simulink model "simBiorreactor_growth"  (R2020b)
settings: Solver=ode45  StartTime=0.0  StopTime=1000  MaxStep=1  RelTol=1e-3  AbsTol=1e-6
undefined symbols (not defined in the file or in its folder): p
settings Model: Creator=nobel  LastModifiedBy=natha

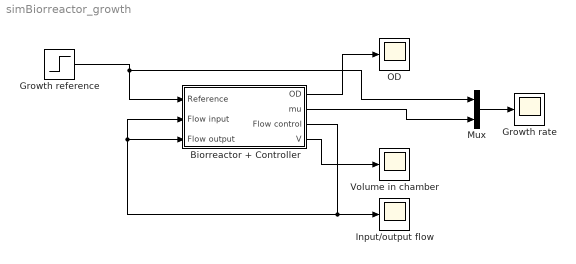
== system simBiorreactor_growth ==
  Biorreactor + Controller : Subsystem
  Growth rate : Scope
  Growth reference : Step  Time=600  Before=0.01  After=0.02  SampleTime=0
  Input/output flow : Scope
  Mux : Mux  Inputs=2
  OD : Scope
  Volume in chamber : Scope
  wires:
  Growth reference/1 -> Mux/1, Biorreactor + Controller/1(Reference)
  Biorreactor + Controller/3(Flow control) -> Input/output flow/1, Biorreactor + Controller/2(Flow input), Biorreactor + Controller/3(Flow output)
  Biorreactor + Controller/1(OD) -> OD/1
  Biorreactor + Controller/4(V) -> Volume in chamber/1
  Mux/1 -> Growth rate/1
  Biorreactor + Controller/2(mu) -> Mux/2

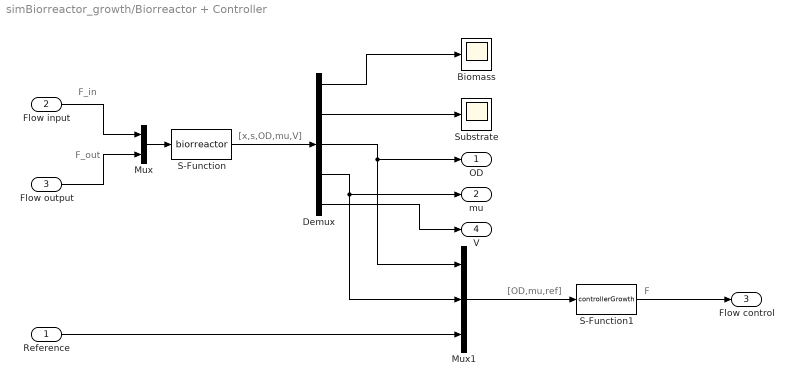
== system simBiorreactor_growth/Biorreactor + Controller ==
  note: F_out
  note: [OD,mu,ref]
  note: F
  note: [x,s,OD,mu,V]
  note: F_in
  Reference : Inport
  Flow input : Inport  Port=2
  Flow output : Inport  Port=3
  Biomass : Scope
  Demux : Demux  Outputs=5
  Mux : Mux  Inputs=2
  Mux1 : Mux  Inputs=3
  S-Function : S-Function  FunctionName=biorreactor  Parameters=[0.1 16 15],p  SFunctionDeploymentMode=off  EnableBusSupport=off
  S-Function1 : S-Function  FunctionName=controllerGrowth  Parameters=p  SFunctionDeploymentMode=off  EnableBusSupport=off
  Substrate : Scope
  OD : Outport
  mu : Outport  Port=2
  Flow control : Outport  Port=3
  V : Outport  Port=4
  wires:
  Demux/4 -> Mux1/2, mu/1
  Demux/3 -> Mux1/1, OD/1
  Reference/1 -> Mux1/3
  S-Function/1 -> Demux/1
  Demux/2 -> Substrate/1
  Mux1/1 -> S-Function1/1
  S-Function1/1 -> Flow control/1
  Demux/1 -> Biomass/1
  Demux/5 -> V/1
  Mux/1 -> S-Function/1
  Flow input/1 -> Mux/1
  Flow output/1 -> Mux/2
